simulink model "nxt_bluetooth"  (R2013b)
settings: Solver=FixedStepDiscrete  SolverMode=SingleTasking  StartTime=0.0  StopTime=inf  FixedStep=balancer_ts  RelTol=1e-3
libraries: legonxtlib x3
settings Model: DataDictionary=mainDict.sldd  ExtModeTrigDuration=2  Creator=mbiesiad  LastModifiedBy=menkh
settings ConfigSet: Description=Use this configuration to communicate between two robots. This robot is the master.
settings OptimizationCC: OptimizeModelRefInitCode=on  LifeSpan=1
settings DebuggingCC: UnderspecifiedInitializationDetection=Simplified  SolverPrmCheckMsg=none  ParameterPrecisionLossMsg=none  SignalLabelMismatchMsg=error  NonBusSignalsTreatedAsBus=error
settings HardwareCC: ProdLargestAtomicInteger=Long  ProdLargestAtomicFloat=Float  ProdEndianess=LittleEndian  ProdHWDeviceType=ARM Compatible->ARM 7
settings RTWCC: SystemTargetFile=realtime.tlc  GenerateMakefile=off  TemplateMakefile=realtime.tmf  Description=Run on Target Hardware  RTWVerbose=off  ProcessScript=realtime_make_rtw_hook
settings STFCustomTargetCC: TargetLibSuffix=.a  GenerateSampleERTMain=on  ERTCustomFileBanners=on  SupportNonInlinedSFcns=off  SupportVariableSizeSignals=on  MATLABClassNameForMDSCustomization=Simulink.SoftwareTarget.ERTCustomization  GRTInterface=off  SystemTargetFile=realtime.tlc
settings ERTTargetCC: CodeReplacementLibrary=ANSI_C  GenerateSampleERTMain=on  ParMdlRefBuildCompliant=off  CompOptLevelCompliant=off  ConcurrentExecutionCompliant=off  CombineOutputUpdateFcns=off  ERTFirstTimeCompliant=off  SupportContinuousTime=on  SupportVariableSizeSignals=on  ModelStepFunctionPrototypeControlCompliant=off  CPPClassGenCompliant=off  ExtModeTransport=1  ExtModeMexFile=ext_serial_win32_comm_no_acks_rtt_byteswap  ExtModeMexArgs=0 1 9600  InlinedParameterPlacement=NonHierarchical  ERTSrcFileBannerTemplate=realtime_code_template.cgt  ERTHdrFileBannerTemplate=realtime_code_template.cgt  ERTDataSrcFileTemplate=realtime_code_template.cgt  ERTDataHdrFileTemplate=realtime_code_template.cgt  ERTCustomFileTemplate=realtime_file_process.tlc

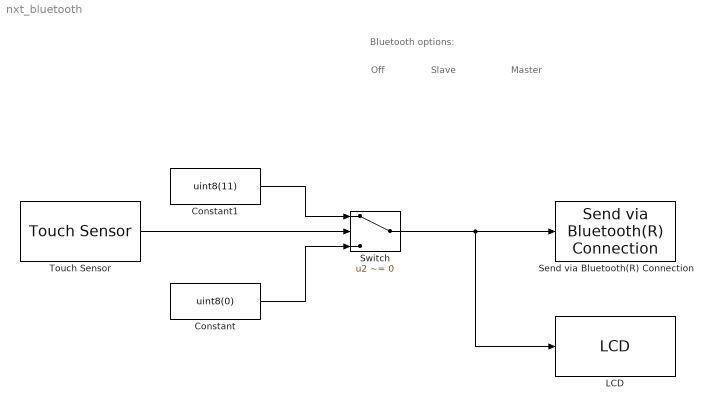
== system nxt_bluetooth ==
  note: Bluetooth options:
  note: Slave
  note: Master
  note: Off
  Constant : Constant  Value=uint8(0)  SampleTime=0.1
  Constant1 : Constant  Value=uint8(11)  SampleTime=0.1
  LCD : legonxtlib/LCD  slcdStr=BT_OUT  slcdLine=1  slcdFormat=Decimal
  Send via Bluetooth(R) Connection : legonxtlib/Send via Bluetooth(R) Connection  mailbox=2
  Switch : Switch  Criteria=u2 ~= 0
  Touch Sensor : legonxtlib/Touch Sensor  portNumber=4  sampleTime=0.1
  wires:
  Constant/1 -> Switch/3
  Switch/1 -> LCD/1, Send via Bluetooth(R) Connection/1
  Touch Sensor/1 -> Switch/2
  Constant1/1 -> Switch/1
